simulink model "EMG_FES2-backup(14-8-2017)"  (R2014a)
settings: Solver=FixedStepDiscrete  StartTime=0.0  StopTime=100  FixedStep=1/aFES.Fs  RelTol=1e-3
InitFcn:
  | if ~exist('aFES','var')
  |   load('afes_param')
  | 
  |    aFES.Fs=1000;
  |    if (~isfield(aFES,'stimCurr'))
  |        aFES.stimCurr=[15,15];
  |    end
  |    aFES.stimFreq=25;
  |    aFES.hand='left';
  | 
  |    %set run number
  |    if (isfield(aFES,'runNum'))
  |          aFES.runNum=aFES.runNum+1;
  |    else
  |          aFES.runNum=1;
  |    end
  | 
  |    %Bias
  |    aFES.wristPosZeroBias=1.8; %e.g: goniometer reading at zeros flexion and extension
  | 
  |    %Set the upper and lower safty limit of the sensor
  |    sensorUpperSafety1=aFES.activeSensorMax+(aFES.activeSensorMax-aFES.activeSensorMin)/4 ;
  |    sensorLowerSafety1=aFES.activeSensorMin-(aFES.activeSensorMax-aFES.activeSensorMin)/4 ;
  | 
  | 
  |    %% Feedback
  |    aFES=emgfes_feedback(aFES,0,0);
  |    aFES.doubleThresh=[0.2,0.4];%Ambrosini double threshold
  | 
  |    %% FIlters
  |    [aFES.EMG_bandpass_b,aFES.EMG_bandpass_a]=butter(5,2*[40,400]/aFES.Fs);
  | 
  |    %% Tracing
  |    aFES.tracing.reflectFeedback =-1;% {1,-1} e.g if the -1, gonirmeter signal will be multiplied by -1.
  |    aFES.tracing.MaxHeightFactor=1;%when >1 scales down the max traceable height. When < 1, scales up the max traceable hieght.
  |    [~,trap_y]=trapezoid4trace();%get the trapezium to be traced
  |    n_z=5;
  |    zero_pad=zeros(n_z*aFES.Fs,1);
  | 
  |    trap_yt=[[0:1/aFES.Fs:((((n_z*aFES.Fs)+2*length(trap_y))/aFES.Fs))-(1/aFES.Fs)]', [zero_pad;trap_y;-trap_y]]; %add time to the trap
  | 
  | end
StopFcn:
  | %save the calibration data but don't apply it
  | aFES.temp.activeSensorMin=calib1_activeSensorMin;
  | aFES.temp.activeSensorMax=calib1_activeSensorMax;
  | 
  | clear calib1_activeSensorMin calib1_activeSensorMax;
  | 
  | %save(['data/afes_data_run',mat2str(aFES.runNum),'.mat'],'aFES','pw_applied','rawProcSignal');
  | save(aFES.fn,'aFES','pw_applied','rawProcSignal');
  | disp('Run data is saved');
  | 
  | disp('Calibration data is updated but not applied. ');
  | disp('To apply it run: aFES.activeSensorMin=aFES.temp.activeSensorMin;  aFES.activeSensorMax=aFES.temp.activeSensorMax; ');
  | 
  | %see if h_keepalife which is use for block event listener attachment object is present and clear it
  | if exist('h_keepalife','var')
  |         clear h_keepalife;
  | end
undefined symbols (not defined in the file or in its folder): analoginput, emgfes_feedback
libraries: dspmtrx3 x4, dspswit3 x3, simulink x2, ScienceStimHasomed_Lib x2, dspinverses x2, daqlib x1
settings Model: Creator=bethel.osuagwu  LastModifiedBy=bethel.osuagwu

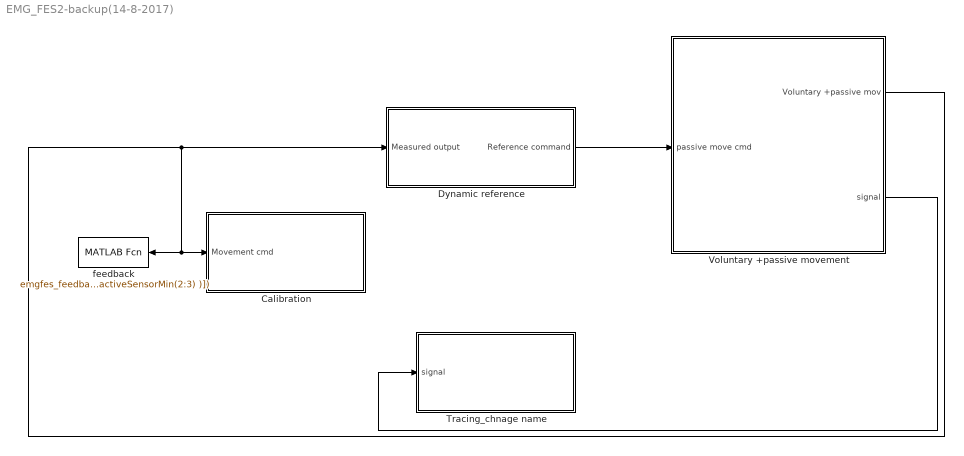
== system EMG_FES2-backup(14-8-2017) ==
  Calibration : Subsystem
  Dynamic reference : Subsystem
  Tracing_chnage name : Subsystem
  Voluntary +passive movement : Subsystem
  feedback : MATLABFcn  MATLABFcn=emgfes_feedback(aFES,[u(1), (u(2:3)'-aFES.activeSensorMin(2:3))./(aFES.activeSensorMax(2:3)-aFES.activeSensorMin(2:3) )])  OutputDimensions=0
  wires:
  Dynamic reference/1(Reference command) -> Voluntary +passive movement/1(passive move cmd)
  Voluntary +passive movement/1(Voluntary +passive mov) -> Dynamic reference/1(Measured output), feedback/1, Calibration/1(Movement cmd)
  Voluntary +passive movement/2(signal) -> Tracing_chnage name/1(signal)

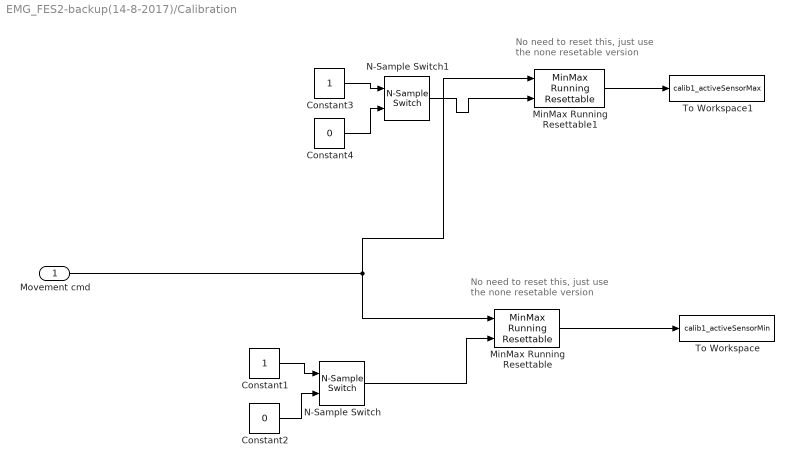
== system EMG_FES2-backup(14-8-2017)/Calibration ==
  note: No need to reset this, just use
      |  the none resetable version
  note: No need to reset this, just use
      |  the none resetable version
  Movement cmd : Inport
  Constant1 : Constant
  Constant2 : Constant  Value=0
  Constant3 : Constant
  Constant4 : Constant  Value=0
  MinMax Running Resettable : simulink/Math Operations/MinMax Running Resettable  Function=min  vinit=inf
  MinMax Running Resettable1 : simulink/Math Operations/MinMax Running Resettable  Function=max  vinit=-inf
  N-Sample Switch : dspswit3/N-Sample Switch  N=10000  reset=off  TriggerType=Rising edge  Ts=-1
  N-Sample Switch1 : dspswit3/N-Sample Switch  N=10000  reset=off  TriggerType=Rising edge  Ts=-1
  To Workspace : ToWorkspace  VariableName=calib1_activeSensorMin  SampleTime=-1
      settings: MaxDataPoints=1
  To Workspace1 : ToWorkspace  VariableName=calib1_activeSensorMax  SampleTime=-1
      settings: MaxDataPoints=1
  wires:
  N-Sample Switch1/1 -> MinMax Running Resettable1/2
  Constant1/1 -> N-Sample Switch/1
  MinMax Running Resettable1/1 -> To Workspace1/1
  MinMax Running Resettable/1 -> To Workspace/1
  N-Sample Switch/1 -> MinMax Running Resettable/2
  Constant2/1 -> N-Sample Switch/2
  Constant3/1 -> N-Sample Switch1/1
  Constant4/1 -> N-Sample Switch1/2
  Movement cmd/1 -> MinMax Running Resettable1/1, MinMax Running Resettable/1

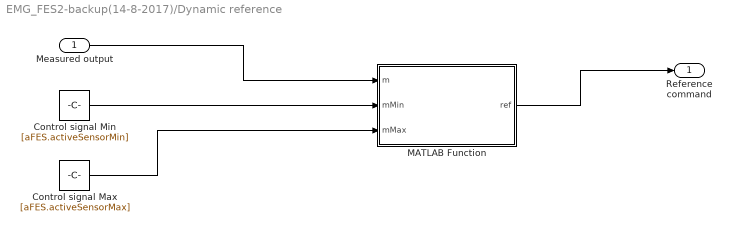
== system EMG_FES2-backup(14-8-2017)/Dynamic reference ==
  Measured output : Inport
  Control signal Max : Constant  Value=[aFES.activeSensorMax]
  Control signal Min : Constant  Value=[aFES.activeSensorMin]
  MATLAB Function : MATLAB Function  TreatAsAtomicUnit=on
  Reference command : Outport
  wires:
  Measured output/1 -> MATLAB Function/1(m)
  MATLAB Function/1(ref) -> Reference command/1
  Control signal Min/1 -> MATLAB Function/2(mMin)
  Control signal Max/1 -> MATLAB Function/3(mMax)

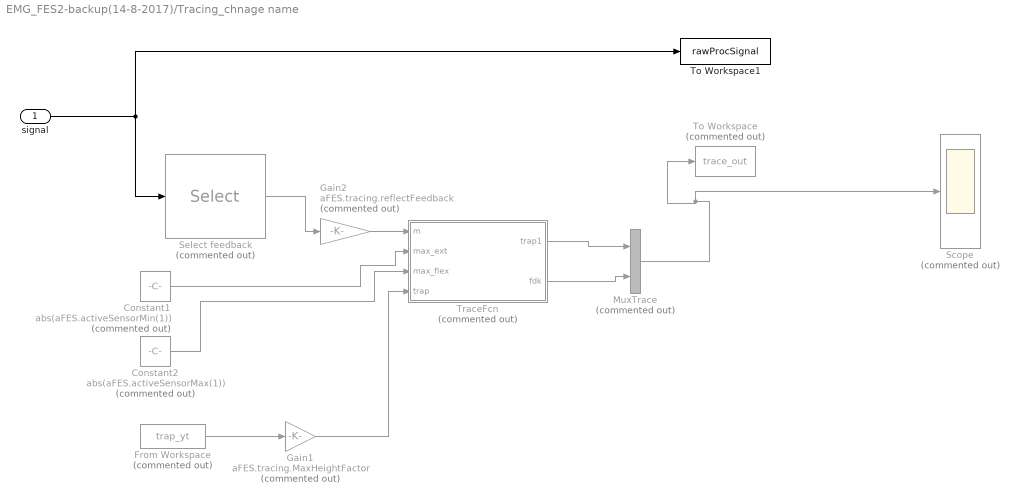
== system EMG_FES2-backup(14-8-2017)/Tracing_chnage name ==
  signal : Inport
  Constant1 : Constant  Commented=on  Value=abs(aFES.activeSensorMin(1))
  Constant2 : Constant  Commented=on  Value=abs(aFES.activeSensorMax(1))
  From Workspace : FromWorkspace  Commented=on  VariableName=trap_yt  SampleTime=1/aFES.Fs  OutputAfterFinalValue=Setting to zero
  Gain1 : Gain  Commented=on  Gain=aFES.tracing.MaxHeightFactor
  Gain2 : Gain  Commented=on  Gain=aFES.tracing.reflectFeedback
  MuxTrace : Mux  Commented=on  Inputs=2
  Scope : Scope  Commented=on
      settings: TimeRange=100  YMin=-2.25  YMax=2  SaveName=ScopeData2
  Select feedback : Selector  Commented=on  InputPortWidth=9  Indices=[7]
  To Workspace : ToWorkspace  Commented=on  VariableName=trace_out  SampleTime=-1
  To Workspace1 : ToWorkspace  VariableName=rawProcSignal  SampleTime=-1
  TraceFcn : MATLAB Function  Commented=on  TreatAsAtomicUnit=on
  wires:
  TraceFcn/1(trap1) -> MuxTrace/1
  MuxTrace/1 -> Scope/1, To Workspace/1
  Gain1/1 -> TraceFcn/4(trap)
  Constant1/1 -> TraceFcn/2(max_ext)
  Constant2/1 -> TraceFcn/3(max_flex)
  signal/1 -> Select feedback/1, To Workspace1/1
  From Workspace/1 -> Gain1/1
  TraceFcn/2(fdk) -> MuxTrace/2
  Select feedback/1 -> Gain2/1
  Gain2/1 -> TraceFcn/1(m)

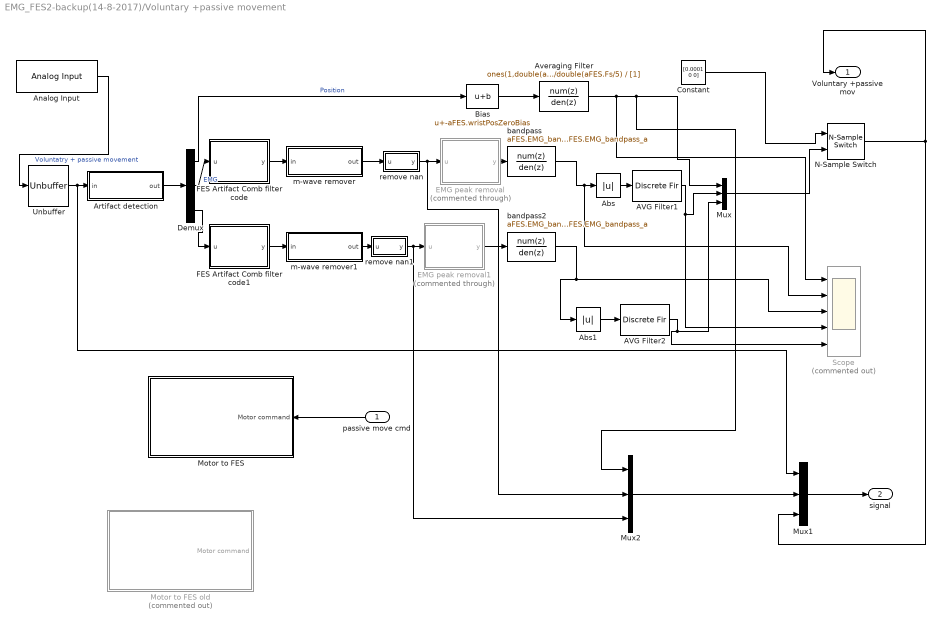
== system EMG_FES2-backup(14-8-2017)/Voluntary +passive movement ==
  passive move cmd : Inport
  " AVG Filter1" : DiscreteFir  Coefficients=ones(1,1000)/1000
  " AVG Filter2" : DiscreteFir  Coefficients=ones(1,1000)/1000
  Abs : Abs
  Abs1 : Abs
  Analog Input : daqlib/Analog Input  AcqMode=0  DeviceMenu=nidaq Dev1 (USB-6341 (BNC))  Device=nidaq Dev1 (USB-6341 (BNC))  ObjConstructor=analoginput('nidaq','Dev1')  SampleRate=1000  ActualRate=1000  SamplesPerFrame=2  InputType=Differential  NChannelsSelected=3  Channels=1$0$$2$#1$1$$2$#1$2$$2$#0$3$$1$#0$4$$1$#0$5$$1$#0$6$$1$#0$7$$1$#  NPorts=1 for all hardware channels  DataType=double
      settings: SignalType=Sample-based
  Artifact detection : Subsystem
  Averaging Filter : DiscreteFilter  Numerator=ones(1,double(aFES.Fs/5))/double(aFES.Fs/5)  Denominator=[1]
  Bias : Bias  Bias=-aFES.wristPosZeroBias
  Constant : Constant  Value=[0.0001 0 0]
  Demux : Demux  Outputs=3
  EMG peak removal : MATLAB Function  Commented=through  TreatAsAtomicUnit=on
  EMG peak removal1 : MATLAB Function  Commented=through  TreatAsAtomicUnit=on
  FES Artifact Comb filter code : MATLAB Function  TreatAsAtomicUnit=on
  FES Artifact Comb filter code1 : MATLAB Function  TreatAsAtomicUnit=on
  Motor to FES : Subsystem
  Motor to FES old : Subsystem  Commented=on
  Mux : Mux  Inputs=3
  Mux1 : Mux  Inputs=3
  Mux2 : Mux  Inputs=3
  N-Sample Switch : dspswit3/N-Sample Switch  N=10  reset=off  TriggerType=Rising edge  Ts=-1
  Scope : Scope  Commented=on  NumInputPorts=5
      settings: YMin=-1~-0.05~-0.075~0~0  YMax=0.75~0.05~0.075~0.007~0.0125
  Unbuffer : Unbuffer  SampleBasedProcessing=Same as frame based
  bandpass : DiscreteFilter  Numerator=aFES.EMG_bandpass_b  Denominator=aFES.EMG_bandpass_a
  bandpass2 : DiscreteFilter  Numerator=aFES.EMG_bandpass_b  Denominator=aFES.EMG_bandpass_a
  m-wave remover : Subsystem
  m-wave remover1 : Subsystem
  remove nan : MATLAB Function  TreatAsAtomicUnit=on
  remove nan1 : MATLAB Function  TreatAsAtomicUnit=on
  Voluntary +passive mov : Outport
  signal : Outport  Port=2
  wires:
  Analog Input/1 -> Unbuffer/1  "Voluntatry + passive movement"
  Demux/1 -> Bias/1  "Position"
  Abs/1 -> " AVG Filter1"/1
  " AVG Filter1"/1 -> Scope/4, Mux/2
  passive move cmd/1 -> Motor to FES/1(Motor command)
  Demux/2 -> FES Artifact Comb filter code/1(u)  "EMG"
  Constant/1 -> N-Sample Switch/1
  N-Sample Switch/1 -> Mux1/3, Voluntary +passive mov/1
  Unbuffer/1 -> Mux1/1, Artifact detection/1(in)
  Bias/1 -> Averaging Filter/1
  Averaging Filter/1 -> Scope/1, Mux2/1, Mux/1
  Abs1/1 -> " AVG Filter2"/1
  " AVG Filter2"/1 -> Scope/5, Mux/3
  Demux/3 -> FES Artifact Comb filter code1/1(u)
  FES Artifact Comb filter code/1(y) -> m-wave remover/1(in)
  EMG peak removal1/1(y) -> bandpass2/1
  Mux/1 -> N-Sample Switch/2
  Artifact detection/1(out) -> Demux/1
  m-wave remover/1(out) -> remove nan/1(u)
  FES Artifact Comb filter code1/1(y) -> m-wave remover1/1(in)
  EMG peak removal/1(y) -> bandpass/1
  bandpass/1 -> Scope/2, Abs/1
  bandpass2/1 -> Abs1/1, Scope/3
  remove nan/1(y) -> Mux2/2, EMG peak removal/1(u)
  remove nan1/1(y) -> Mux2/3, EMG peak removal1/1(u)
  m-wave remover1/1(out) -> remove nan1/1(u)
  Mux1/1 -> signal/1
  Mux2/1 -> Mux1/2

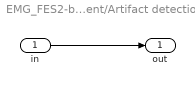
== system EMG_FES2-backup(14-8-2017)/Voluntary +passive movement/Artifact detection ==
  in : Inport
  out : Outport
  wires:
  in/1 -> out/1

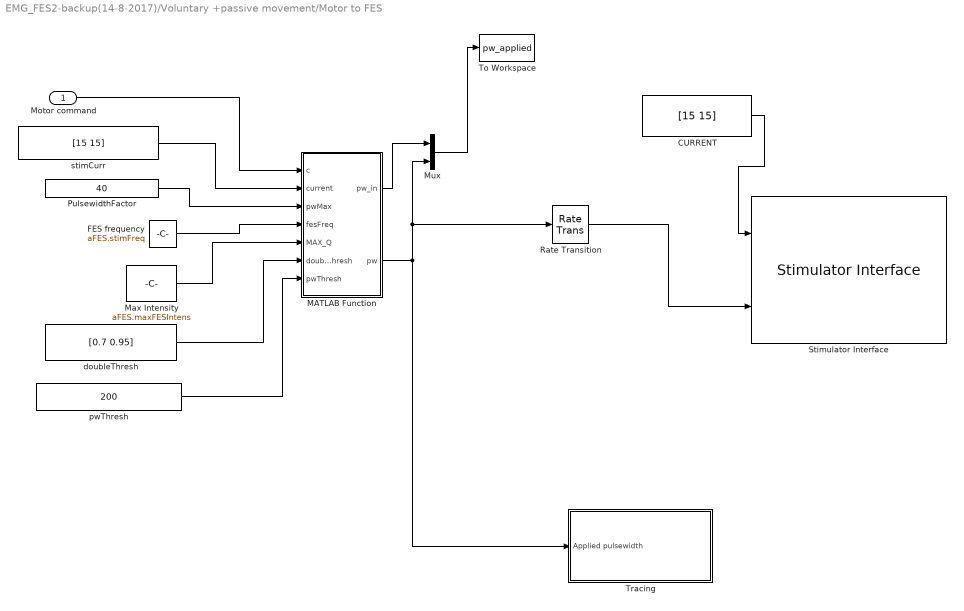
== system EMG_FES2-backup(14-8-2017)/Voluntary +passive movement/Motor to FES ==
  Motor command : Inport
  CURRENT : Constant  Value=[15 15]
  FES frequency : Constant  Value=aFES.stimFreq
  MATLAB Function : MATLAB Function  TreatAsAtomicUnit=on
  Max Intensity : Constant  Value=aFES.maxFESIntens
  Mux : Mux  Inputs=2
  PulsewidthFactor : Constant  Value=40
  Rate Transition : RateTransition
  Stimulator Interface : ScienceStimHasomed_Lib/Stimulator Interface  Ts=33/aFES.Fs  com_port=COM9  channelstim=[1,2]  tsone=round((1/aFES.stimFreq)*1000)  tstwo=5  channellf=[]  nfactor=[]  outflag=off  dtflag=off
  To Workspace : ToWorkspace  VariableName=pw_applied  SampleTime=-1
  Tracing : Subsystem
  doubleThresh : Constant  Value=[0.7 0.95]
  pwThresh : Constant  Value=200
  stimCurr : Constant  Value=[15 15]
  wires:
  CURRENT/1 -> Stimulator Interface/1
  Motor command/1 -> MATLAB Function/1(c)
  MATLAB Function/2(pw) -> Tracing/1(Applied pulsewidth), Mux/2, Rate Transition/1
  Rate Transition/1 -> Stimulator Interface/2
  stimCurr/1 -> MATLAB Function/2(current)
  Max Intensity/1 -> MATLAB Function/5(MAX_Q)
  doubleThresh/1 -> MATLAB Function/6(doubleThresh)
  MATLAB Function/1(pw_in) -> Mux/1
  Mux/1 -> To Workspace/1
  pwThresh/1 -> MATLAB Function/7(pwThresh)
  FES frequency/1 -> MATLAB Function/4(fesFreq)
  PulsewidthFactor/1 -> MATLAB Function/3(pwMax)

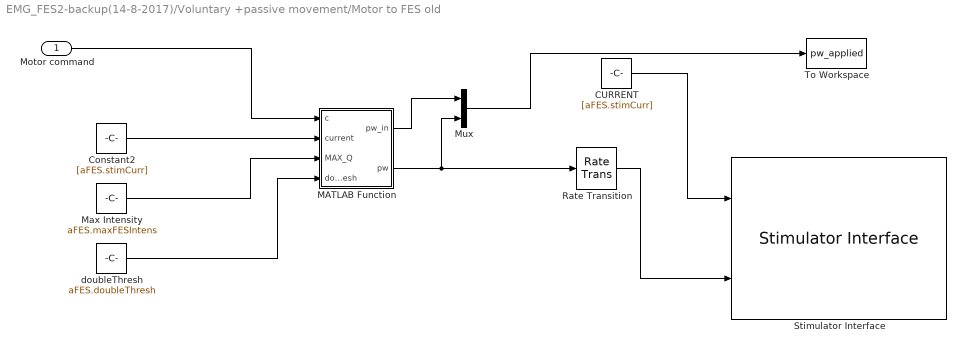
== system EMG_FES2-backup(14-8-2017)/Voluntary +passive movement/Motor to FES old ==
  Motor command : Inport
  CURRENT : Constant  Value=[aFES.stimCurr]
  Constant2 : Constant  Value=[aFES.stimCurr]
  MATLAB Function : MATLAB Function  TreatAsAtomicUnit=on
  Max Intensity : Constant  Value=aFES.maxFESIntens
  Mux : Mux  Inputs=2
  Rate Transition : RateTransition
  Stimulator Interface : ScienceStimHasomed_Lib/Stimulator Interface  Ts=33/aFES.Fs  com_port=COM9  channelstim=[1,2]  tsone=round((1/aFES.stimFreq)*1000)  tstwo=5  channellf=[]  nfactor=[]  outflag=off  dtflag=off
  To Workspace : ToWorkspace  VariableName=pw_applied  SampleTime=-1
  doubleThresh : Constant  Value=aFES.doubleThresh
  wires:
  Mux/1 -> To Workspace/1
  MATLAB Function/1(pw_in) -> Mux/1
  doubleThresh/1 -> MATLAB Function/4(doubleThresh)
  Max Intensity/1 -> MATLAB Function/3(MAX_Q)
  Constant2/1 -> MATLAB Function/2(current)
  Rate Transition/1 -> Stimulator Interface/2
  MATLAB Function/2(pw) -> Rate Transition/1, Mux/2
  Motor command/1 -> MATLAB Function/1(c)
  CURRENT/1 -> Stimulator Interface/1

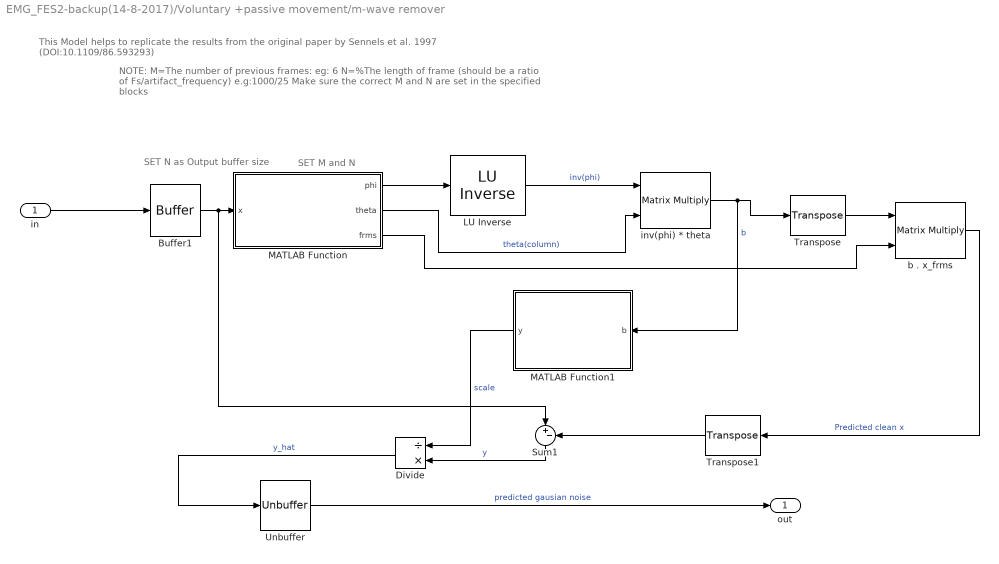
== system EMG_FES2-backup(14-8-2017)/Voluntary +passive movement/m-wave remover ==
  note: NOTE:
      | M=The number of previous frames: eg: 6
      | N=%The length of frame (should be a ratio of Fs/artifact_frequency) e.g:1000/25
      | Make sure the correct M and N are set in the specified blocks
  note: SET N as Output
      | buffer size
  note: SET M and N
  note: This Model helps to replicate the results from the original paper by Sennels et al. 1997 (DOI:10.1109/86.593293)
  in : Inport
  " LU Inverse" : dspinverses/ LU Inverse
  Buffer1 : Buffer  N=40  TreatMby1Signals=One channel
  Divide : Product  Inputs=/*
  MATLAB Function : MATLAB Function  TreatAsAtomicUnit=on
  MATLAB Function1 : MATLAB Function  TreatAsAtomicUnit=on
  Sum1 : Sum  Inputs=|+-
  Transpose : dspmtrx3/Transpose  Hermitian=off  overflowFlag=off
  Transpose1 : dspmtrx3/Transpose  Hermitian=off  overflowFlag=off
  Unbuffer : Unbuffer  SampleBasedProcessing=Same as frame based
  b . x_frms : Product  Multiplication=Matrix(*)
  inv(phi) * theta : Product  Multiplication=Matrix(*)
  out : Outport
  wires:
  Buffer1/1 -> Sum1/1, MATLAB Function/1(x)
  MATLAB Function/1(phi) -> " LU Inverse"/1
  MATLAB Function/2(theta) -> inv(phi) * theta/2  "theta(column)"
  " LU Inverse"/1 -> inv(phi) * theta/1  "inv(phi)"
  inv(phi) * theta/1 -> MATLAB Function1/1(b), Transpose/1  "b"
  Unbuffer/1 -> out/1  "predicted gausian noise"
  MATLAB Function/3(frms) -> b . x_frms/2
  Transpose/1 -> b . x_frms/1
  b . x_frms/1 -> Transpose1/1  "Predicted clean x"
  Transpose1/1 -> Sum1/2
  Sum1/1 -> Divide/2  "y"
  MATLAB Function1/1(y) -> Divide/1  "scale"
  Divide/1 -> Unbuffer/1  "y_hat"
  in/1 -> Buffer1/1

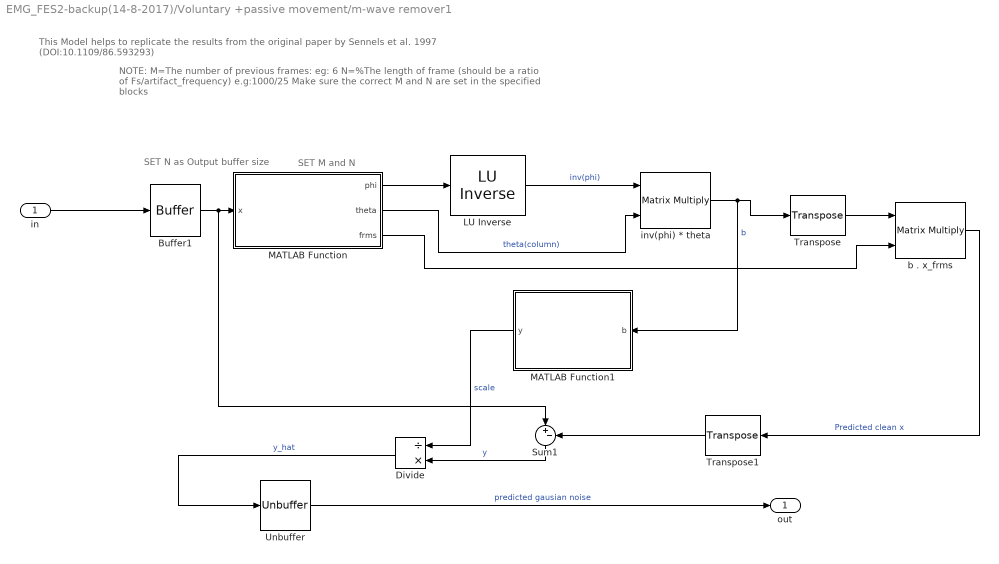
== system EMG_FES2-backup(14-8-2017)/Voluntary +passive movement/m-wave remover1 ==
  note: NOTE:
      | M=The number of previous frames: eg: 6
      | N=%The length of frame (should be a ratio of Fs/artifact_frequency) e.g:1000/25
      | Make sure the correct M and N are set in the specified blocks
  note: SET N as Output
      | buffer size
  note: SET M and N
  note: This Model helps to replicate the results from the original paper by Sennels et al. 1997 (DOI:10.1109/86.593293)
  in : Inport
  " LU Inverse" : dspinverses/ LU Inverse
  Buffer1 : Buffer  N=80  TreatMby1Signals=One channel
  Divide : Product  Inputs=/*
  MATLAB Function : MATLAB Function  TreatAsAtomicUnit=on
  MATLAB Function1 : MATLAB Function  TreatAsAtomicUnit=on
  Sum1 : Sum  Inputs=|+-
  Transpose : dspmtrx3/Transpose  Hermitian=off  overflowFlag=off
  Transpose1 : dspmtrx3/Transpose  Hermitian=off  overflowFlag=off
  Unbuffer : Unbuffer  SampleBasedProcessing=Same as frame based
  b . x_frms : Product  Multiplication=Matrix(*)
  inv(phi) * theta : Product  Multiplication=Matrix(*)
  out : Outport
  wires:
  Buffer1/1 -> Sum1/1, MATLAB Function/1(x)
  MATLAB Function/1(phi) -> " LU Inverse"/1
  MATLAB Function/2(theta) -> inv(phi) * theta/2  "theta(column)"
  " LU Inverse"/1 -> inv(phi) * theta/1  "inv(phi)"
  inv(phi) * theta/1 -> MATLAB Function1/1(b), Transpose/1  "b"
  Unbuffer/1 -> out/1  "predicted gausian noise"
  MATLAB Function/3(frms) -> b . x_frms/2
  Transpose/1 -> b . x_frms/1
  b . x_frms/1 -> Transpose1/1  "Predicted clean x"
  Transpose1/1 -> Sum1/2
  Sum1/1 -> Divide/2  "y"
  MATLAB Function1/1(y) -> Divide/1  "scale"
  Divide/1 -> Unbuffer/1  "y_hat"
  in/1 -> Buffer1/1

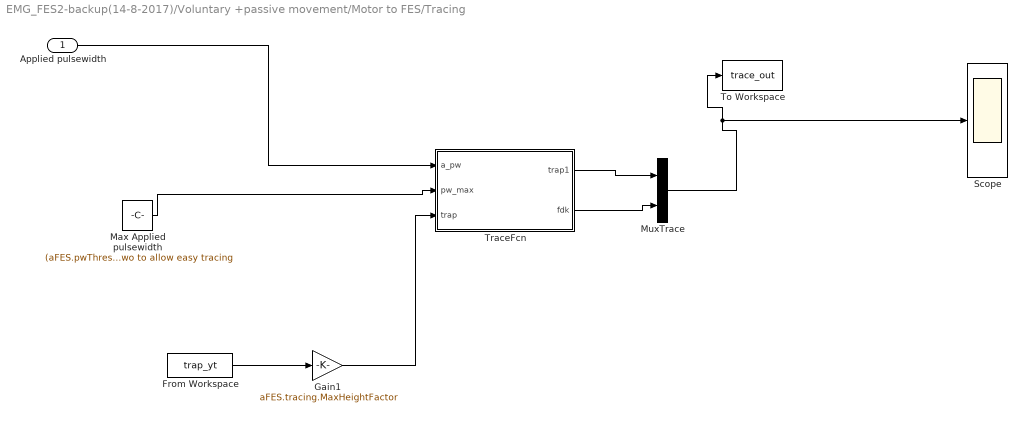
== system EMG_FES2-backup(14-8-2017)/Voluntary +passive movement/Motor to FES/Tracing ==
  Applied pulsewidth : Inport
  From Workspace : FromWorkspace  VariableName=trap_yt  SampleTime=1/aFES.Fs  OutputAfterFinalValue=Setting to zero
  Gain1 : Gain  Gain=aFES.tracing.MaxHeightFactor
  Max Applied pulsewidth : Constant  Value=(aFES.pwThresh+aFES.pwFactor*max(aFES.activeSensorMax(2:3)))/2 %we devide by two to allow easy tracing
  MuxTrace : Mux  Inputs=2
  Scope : Scope
      settings: TimeRange=100  YMin=-2.25  YMax=2  SaveName=ScopeData2
  To Workspace : ToWorkspace  VariableName=trace_out  SampleTime=-1
  TraceFcn : MATLAB Function  TreatAsAtomicUnit=on
  wires:
  TraceFcn/1(trap1) -> MuxTrace/1
  MuxTrace/1 -> To Workspace/1, Scope/1
  Gain1/1 -> TraceFcn/3(trap)
  Max Applied pulsewidth/1 -> TraceFcn/2(pw_max)
  From Workspace/1 -> Gain1/1
  TraceFcn/2(fdk) -> MuxTrace/2
  Applied pulsewidth/1 -> TraceFcn/1(a_pw)

== matlab function EMG_FES2-backup(14-8-2017)/Dynamic reference/MATLAB Function ==
  data: m input; mMin input; ref output; mMax input
function ref   = fcn(m,mMin,mMax)
%#codegen
%m(1)=position/force, extension should have negative values while flexion
%have positiove values and 0 is neutral
%m(2:3) measure of ext. EMG and Flex EMG power respectively (i.e.
%m(3)->extension and m(3)->flexion
%
%mMin and mMax are the calibration min and max resp. for m values
%
%
%
%SeSsions maked as modules can be removed without causing too much harm to
%the system, removing them just removes their minor function which does not
%affect the main system
%
%
persistent t_blocking ref_mem act_chnl_mem act_mem;
% act_chnl_mem ={0:3}. Tells us which 'vitual' channel is on. 0:none;
% 1:extension; 2:flexion; 3:tenodesis grip; 4:tenodesis release; 5:both
% flexion and extension

%assert(m<=3);

%% General parameters 

%These should be determin at the starte of every test and should be input to the fucntion
mMaxVolPercent=[1;0.9999999;0.999999];%The percentage of max voluntary value to be used as the actuall Max. E.g 0.5, means  50% of mMax is used as the actual mMax while a value of 1 means to use full mMax as mMax
mMax_=mMax.*mMaxVolPercent;%Rescale mMax

wristMax=mMax_(1);
wristMin=mMin(1);

pFlexRefMax=mMax_(3);
pFlexRefMin=mMin(3);

pExtRefMax=mMax_(2);
pExtRefMin=mMin(2);

tenodesisON=[0;0];%1=allow tenodesis; 0=No tenodesis: tenodesisON(1) for tenodesis grip. tenodesisON(2) for tenodesis release

wristExtTenoPerc =0.95;% The percentage of max wrist extension at which forced(i.e based only on wrist) tenodesis grip should be activated
wristFlexTenoPerc =0.97;%The percentage of max wrist flexion at which forced (i.e based only on wrist) tenodesis release should be activated

extTenoPerc =0.80;% The percentage of max wrist extension at which activated(i.e based on both finger and wrist, Tenodesis proper) tenodesis grip should be activated
flexTenoPerc =0.80;%The percentage of max wrist flexion at which activated (i.e based on both finger and wrist Tenodesis proper) tenodesis release should be activated

act_opposeLowerPerc=0.7;%{1= no lowering of activation threshold, 0=lower activation threshold to zero}the percentage to lower the activation of an opposing movement to give it a chance to activate

%calculate the activation threshold as a set percentage above the the
%minimun signal
act_thresh_ext=mMin(2)+0.05*mMin(2);
act_thresh_flex=mMin(3)+0.05*mMin(3);

%%Add small activation based on goniometer position. BUT FOR BETTER CONTROL, TURN THIS OFF IF
%%FES INTENSITY IS HIGH TO PRODUCE LARGE MOVEMENT \KODE*~#1.
wristActSuppON=[0;0];%{see \KODE *~#1)true to turn ON supplimentary activation when the wrist is moved above threshold:: wristActSuppON(1)=>ext; wristActSuppON(2)=>flex
wristActThresh =[wristMin;wristMax]*0.05; %the activation threshold for wrist movement

%Blocking window
oppositeRefracWin =1000;%The number of samples for which to refrain from imidiate opposite movement



%% Begin
if(isempty(t_blocking))    
   ref=m(2:3);%Make the current reference
   ref_mem=ref;
   t_blocking=0;
   act_chnl_mem=0;
   act_mem=0;
   return;
end

%update blocking timing
if t_blocking 
    if t_blocking>=oppositeRefracWin %refractory period of samples
        t_blocking=0;
    else
        t_blocking=t_blocking+1;
    end
end


%% Compute relative power
m(3)=(m(3)-pFlexRefMin)/(pFlexRefMax-pFlexRefMin);
m(2)=(m(2)-pExtRefMin)/(pExtRefMax-pExtRefMin);



%% Compute channel selection parameters
wristFlex=0;
wristExt=0;
tenoGras=0;
tenoRelease=0;
wristActSupp=[0;0];
if m(1)>0 
    wristFlex=1;%flex
    act_thresh_ext=act_thresh_ext*act_opposeLowerPerc;% lower the activation threshold of extension when the wrist is flex( Note that this might have been done by an external block):
    
    %%wrist position adds a bit of activation for flexion
    if m(1)>wristActThresh(2) && wristActSuppON(2)
        wristActSupp(2)=m(3)*0.4+0.2;
    end
    
    if(tenodesisON(2))
        if m(1)>wristMax*wristFlexTenoPerc 
            tenoRelease=1;   
        end
    end
    
else
    wristExt=1;%extension
    act_thresh_flex=act_thresh_flex*act_opposeLowerPerc ;% lower the activation threshold of flexion when the wrist extended: (Note that this might have been done by an external block)
    
    %%wrist position adds a bit of activation for extension
    if m(1)<wristActThresh(1) && wristActSuppON(1)
        wristActSupp(1)=m(2)*0.4+0.2;
    end
    
    if m(1)<wristMin*wristExtTenoPerc %TODO: check ik if (tenodesisON(1)==1
        tenoGras=1;
    end
 
end

%% Are current values greater than their thresh hold
pFlex=0;
if m(3)>act_thresh_flex
    pFlex=1;
end

pExt=0;
if m(2)>act_thresh_ext
    pExt=1;
end


%% Classify flexion and extension
isFlex=double(m(2)<m(3));

isExt=1-isFlex;
if(wristExt && pFlex)
    %So the wrist is extended but the fingers are closing
    isFlex=1; %reinforce that flexion should be on
end
if(wristFlex && pExt)
    %so the writs is flexed but the fingers are opening
    isExt=1;%reinforce that extension should be on
end

%Total flexion
isFlex=isFlex+pFlex+wristFlex;
%Total extension
isExt=isExt+pExt+wristExt;


%% Tenodesis proper (fingers and wrists)
if (wristFlex && m(1)>wristMax*flexTenoPerc && 1.5*m(2)>m(3)) && tenodesisON(2)
    %This is another way to turn on tenodesis release
    tenoRelease=tenoRelease+1;
end

if(wristExt && m(1)<wristMin*extTenoPerc && 1.5*m(3)>m(2)) && tenodesisON(1)
    %This is another way to turn on tenodesis grip
    tenoGras=tenoGras+1;
end


%% Compute ref
if tenoGras && tenodesisON(1)%i.e Tenodesis grip
    ref=m(2:3);% +wristActSupp;
    ref(2)=ref(2) + ref(2)*tenoGras*0.5; %cheat for flexion by the magnitude of the tenoGras
    act_chnl=3; %See header for the meaning of activated channels
elseif tenoRelease && tenodesisON(2)%i.e Tenodesis release
    ref=m(2:3);%+wristActSupp;
    ref(1)=ref(1) + ref(1)*tenoRelease*0.5; %cheat for flexion by the magnitude of the tenoRelease
    act_chnl=4; %See header for the meaning of activated channels
elseif isFlex>isExt
    ref=[0;m(3)];
    ref(2)=ref(2)+wristActSupp(2);
    act_chnl=2;
elseif isExt>isFlex
    ref=[m(2);0];
    ref(1)=ref(1)+wristActSupp(1);
    act_chnl=1;
elseif isExt && isFlex && isExt==isFlex
    ref=m(2:3);%+wristActSupp;
    act_chnl=5;
else   
    ref=[0;0];
    act_chnl=0;
end
act=sum(ref);   

%% Check if we can block activation
%%implements blocking of immediate opposite movement
if ~t_blocking || act_chnl==act_chnl_mem && act>act_mem% The operator precidence here should lead to the correct operation
    t_blocking=1;% start blocking of further imidiate opposite change
else
    ref=ref_mem; 
end


%% Save to mem
if(ref(1)~=ref_mem(1) || ref(2)~=ref_mem(2))
    act_mem=act;
    act_chnl_mem=act_chnl;
    ref_mem=ref;
    
end

== matlab function EMG_FES2-backup(14-8-2017)/Voluntary +passive movement/FES Artifact Comb filter code ==
  data: u input; y output
function y  = fcn(u)
%#codegen

persistent u_mem;
fes_freq=25;%FES frequency
Fs=1000;%EMG/data samplerate
K=40;%round(Fs/fes_freq); %Comb filter order = (1/fes_freq)*Fs
a=-1;%{-1 to 0}
if isempty(u_mem)
    u_mem=zeros(K,1);
end





%% Comb filtering
% Forward comb
y=u+ a*u_mem(1);



u_mem(1:end-1)=u_mem(2:end);
u_mem(end)=u;



end





%

== matlab function EMG_FES2-backup(14-8-2017)/Voluntary +passive movement/Motor to FES/MATLAB Function ==
  data: pw_in output; c input; current input; pw output; pwMax input; fesFreq input; MAX_Q input; doubleThresh input; pwThresh input
function [pw_in,pw] = fcn(c,current,pwMax,fesFreq,MAX_Q,doubleThresh,pwThresh)
%#codegen
% c is the controller output
% current is a vector(1 ele/chnl) of FES current in milliamps
% pwMax is the max pulsewidth 
% fesFreq is the FES frequency
% MAX_Q= eg.5000;%maxmum FES intensity =current x pulsewidth *freq
% doubleThresh {[OFF thresh; ON thresh]}is the double thresh similer to that by Ambrosini
% pwThresh is the starting pulsewidth once activation reaches
%threshold
persistent  FES_ON pw_smooth;


if isempty(pw_smooth)
    %c_mem=zeros(30,2);
    FES_ON=[0;0];
    pw_smooth=[0;0];
    
end


%% (Module) Avoid spikes in Stimulation
% if false
% c(dcdt>0.5)=median(c_mem);
% %upadte memory of controller output
%  c_mem(1:end-1,:)=c_mem(2:end,:);
%  c_mem(end,:)=c;
% end

%compute pulsewidth
if(doubleThresh(2))
    pw=[0;0];
    for chni=1:2
        if FES_ON(chni) %If the channel is ON, check if it has dropped below first double thresh
            if c(chni)<doubleThresh(1)%If the channel has dropped below the first thresh, then turn it OFF
                pw(chni)=0;
                FES_ON(chni)=0;
            else %But if the channel is still above the OFF thresh, then proportionally set the pw
                %pw(chni)=200+c(chni)*30;%
                pw(chni)=pwThresh+c(chni)*pwMax;
                FES_ON(chni)=1;
            end
        else %But is the channel currently OFF, Check if it has activation above ON thresh
            if c(chni)>doubleThresh(2)% If the activation is above ON thresh,then proportionally set the pw
                %pw(chni)=200+c(chni)*30;%
                pw(chni)=pwThresh+c(chni)*pwMax;
                FES_ON(chni)=1;
            else %but if it is still under the ON thresh, make sure that it is set to off
                pw(chni)=0;
                FES_ON(chni)=0;
            end
        end
    end
    
else %Double threshold is disabled, need to proportionally set pw
    pw=(c).*pwMax;%OR %pw=pwThresh+(c).*pwMax;
    
    
    
    %pw(pw<0)=0;
    %pw(pw>50)=pw(pw>50)+10;%add a bias
    pw(pw<50)=0;
end

%% Limit max Intensity of FES
q=current.*pw*fesFreq;
q_=q>MAX_Q;
for nq=1:length(q_)
    if q_(nq)
        pw(nq)=MAX_Q/(current(nq)*fesFreq);
        'Motor to FES: limits [ch,pulsewidth_limit]'
        [nq pw(nq)]
    end
end

%% The estimated pw is essentially our input pw
pw_in=pw;% If no further modification below, then pw_in==pw


%% (Module)Controller output based change in stimulation for opposing movement assistance



%% (Module)Error based change in stimulation for opposing movement assistance


%% (Module) Smoothness controller for pw
pw_step=0.1;%(TODO: should be a function of max pw and samplerate)allowed positive step chnage per sample
pw=abs(pw_smooth+sign(pw-pw_smooth)*pw_step); %the abs here is fine as far as the step size is small(e.g <5)
%pw(pw<pw_step)=0;NOTE open this 
pw_smooth=pw;
%-----------------------------

== matlab function EMG_FES2-backup(14-8-2017)/Voluntary +passive movement/m-wave remover/MATLAB Function ==
  data: x input; phi output double; theta output; frms output
function [phi,theta,frms] = fcn(x)
%#codegen
persistent t_sample phi_mem  frms_mem ;

%General param
M=6; %The number of previous frames 
N=40; %The length of frame (should be a ratio of Fs/artifact_frequency)

% Performance parameter
freshPhi =1;% when =1:recompute phi(covariance matix) all the phi; when =0:update phi with only new values

if isempty(t_sample)
    t_sample=0;
    frms_mem=zeros(M,N);
    
    phi_mem=zeros(M,M);
end
t_sample=t_sample+1;

%make x a row vector
x=x';


%% compute phi
frms=frms_mem;
%equ 7 and 8
if(freshPhi)
    % compute phi fresh all the time
    phi=(frms*frms');
else
    %we can compute only the required column (first) and row (first)of phi
    %matrix and push the new values into phi
    phi_mem(2:end,2:end)=phi_mem(1:end-1,1:end-1);
    phi_mem(1,:)=frms(1,:)*frms';
    phi_mem(:,1)=phi_mem(1,:)';
    %phi-phi_mem
    phi=phi_mem;
end


%% compute theta
theta=(x*frms')';
%t_sample
%if t_sample==15
%    y=4;
%end


%% update frame
frms_mem(2:end,:)=frms_mem(1:end-1,:);
frms_mem(1,:)=x;

== matlab function EMG_FES2-backup(14-8-2017)/Voluntary +passive movement/FES Artifact Comb filter code1 ==
  data: u input; y output
function y  = fcn(u)
%#codegen

persistent u_mem;
fes_freq=25;%FES frequency
Fs=1000;%EMG/data samplerate
K=40;%round(Fs/fes_freq); %Comb filter order = (1/fes_freq)*Fs
a=-1;%{-1 to 0}
if isempty(u_mem)
    u_mem=zeros(K,1);
end





%% Comb filtering
% Forward comb
y=u+ a*u_mem(1);



u_mem(1:end-1)=u_mem(2:end);
u_mem(end)=u;
end





%

== matlab function EMG_FES2-backup(14-8-2017)/Voluntary +passive movement/EMG peak removal1 ==
  data: u input; y output
function y  = fcn(u)
%#codegen
%peak removal
peak_thresh=0.5;
dmdt_thresh=0.3;
blocking_win=50;
persistent u_mem t_;
if isempty(u_mem)
    u_mem=zeros(1000,1);
    t_=0;
end

if (dmdt_thresh<abs(u)-abs(u_mem(end))&& t_==0)%if the change in value to too large  then block with no stats
    t_=1;
else   
    if((abs(u)>peak_thresh || dmdt_thresh<abs(u)-abs(u_mem(end))) && t_==0) %detect high amplitude,peak, and start blocking
        if(abs(u)>std(u_mem))
            t_=1;
        end
    end

    
end


if t_
    u=0;%block
   t_=t_+1;
end
if(t_==blocking_win) %stop blocking after n samples
    t_=0; 
end

u_mem(1:end-1)=u_mem(2:end);
u_mem(end)=u;
y=u;
end





%

== matlab function EMG_FES2-backup(14-8-2017)/Voluntary +passive movement/EMG peak removal ==
  data: u input; y output
function y  = fcn(u)
%#codegen
%peak removal
peak_thresh=0.5;
dmdt_thresh=0.3;
blocking_win=50;
persistent u_mem t_;
if isempty(u_mem)
    u_mem=zeros(1000,1);
    t_=0;
end

if (dmdt_thresh<abs(u)-abs(u_mem(end))&& t_==0)%if the change in value to too large  then block with no stats
    t_=1;
else   
    if((abs(u)>peak_thresh || dmdt_thresh<abs(u)-abs(u_mem(end))) && t_==0) %detect high amplitude,peak, and start blocking
        if(abs(u)>std(u_mem))
            t_=1;
        end
    end

    
end


if t_
    u=0;%block
   t_=t_+1;
end
if(t_==blocking_win) %stop blocking after n samples
    t_=0; 
end

u_mem(1:end-1)=u_mem(2:end);
u_mem(end)=u;
y=u;
end





%

== matlab function EMG_FES2-backup(14-8-2017)/Voluntary +passive movement/remove nan ==
  data: u input; y output
function y  = fcn(u)
%#codegen

y=u;
if isnan(y)
    y=0;
end





%

== matlab function EMG_FES2-backup(14-8-2017)/Voluntary +passive movement/remove nan1 ==
  data: u input; y output
function y  = fcn(u)
%#codegen

y=u;
if isnan(y)
    y=0;
end





%

== matlab function EMG_FES2-backup(14-8-2017)/Voluntary +passive movement/m-wave remover/MATLAB Function1 ==
  data: b input; y output
function y = fcn(b)
%#codegen


y = sqrt(1+sum(b.^2));
%       OR
%y = (1+sum(b));%approximated for speed

== matlab function EMG_FES2-backup(14-8-2017)/Voluntary +passive movement/m-wave remover1/MATLAB Function ==
  data: x input; phi output double; theta output; frms output
function [phi,theta,frms] = fcn(x)
%#codegen
persistent t_sample phi_mem  frms_mem ;

%General param
M=6; %The number of previous frames 
N=80; %The length of frame (should be a ratio of Fs/artifact_frequency)

% Performance parameter
freshPhi =1;% when =1:recompute phi(covariance matix) all the phi; when =0:update phi with only new values

if isempty(t_sample)
    t_sample=0;
    frms_mem=zeros(M,N);
    
    phi_mem=zeros(M,M);
end
t_sample=t_sample+1;

%make x a row vector
x=x';


%% compute phi
frms=frms_mem;
%equ 7 and 8
if(freshPhi)
    % compute phi fresh all the time
    phi=(frms*frms');
else
    %we can compute only the required column (first) and row (first)of phi
    %matrix and push the new values into phi
    phi_mem(2:end,2:end)=phi_mem(1:end-1,1:end-1);
    phi_mem(1,:)=frms(1,:)*frms';
    phi_mem(:,1)=phi_mem(1,:)';
    %phi-phi_mem
    phi=phi_mem;
end


%% compute theta
theta=(x*frms')';
%t_sample
%if t_sample==15
%    y=4;
%end


%% update frame
frms_mem(2:end,:)=frms_mem(1:end-1,:);
frms_mem(1,:)=x;

== matlab function EMG_FES2-backup(14-8-2017)/Voluntary +passive movement/m-wave remover1/MATLAB Function1 ==
  data: b input; y output
function y = fcn(b)
%#codegen


y = sqrt(1+sum(b.^2));
%       OR
%y = (1+sum(b));%approximated for speed

== matlab function EMG_FES2-backup(14-8-2017)/Tracing_chnage name/TraceFcn ==
  data: m input; max_ext input; max_flex input; trap input; trap1 output; fdk output
function [trap1,fdk]    = fcn(m,max_ext,max_flex,trap)
%#codegen
%coder.extrinsic('plot','hold');
% persistent ts;
% if isempty(ts)
%     ts=0;
%     %m_mem=zeros(10*1000,1);
% end
%m_mem(1:end-1)=m_mem(2:end);
%m_mem(end)=m(1);

%scale extension
if(m(1)>0)
    m(1)=m(1)/max_ext;
elseif m(1)<0
    m(1)=m(1)/max_flex;
end
    
%ts=ts+1;
 trap1=trap;
 
 fdk=m(1);
 
%stopSingnal=0;
%  if(ts==length(trap))
%      stopSingnal=1;
%  end

== matlab function EMG_FES2-backup(14-8-2017)/Voluntary +passive movement/Motor to FES old/MATLAB Function ==
  data: pw_in output; c input; current input; pw output; MAX_Q input; doubleThresh input
function [pw_in,pw] = fcn(c,current,MAX_Q,doubleThresh)
%#codegen
% c is the controller output
% dcdt is the derivative of c
%MAX_Q= eg.5000;%maxmum intensity =current x pulsewidth
persistent  FES_ON pw_smooth;

pMax=300;
if isempty(pw_smooth)
    %c_mem=zeros(30,2);
    FES_ON=[0;0];
    pw_smooth=[0;0];
end


%% (Module) Avoid spikes in Stimulation
% if false
% c(dcdt>0.5)=median(c_mem);
% %upadte memory of controller output
%  c_mem(1:end-1,:)=c_mem(2:end,:);
%  c_mem(end,:)=c;
% end

%compute pulsewidth
if(doubleThresh(2))
    pw=[0;0];
    for chni=1:2
        if FES_ON(chni)
            if c(chni)<doubleThresh(1)
                pw(chni)=0;
                FES_ON(chni)=0;
            else
                pw(chni)=200+c(chni).*30;
                FES_ON(chni)=1;
            end
        else %it is currently off
            if c(chni)>doubleThresh(2)
                pw(chni)=200+c(chni).*30;
                FES_ON(chni)=1;
            else
                pw(chni)=0;
                FES_ON(chni)=0;
            end
        end
    end
    
else
    pw=(c).*pMax;
    pw(pw<0)=0;
    %pw(pw>50)=pw(pw>50)+10;%add a bias
    pw(pw<50)=0;
end

%% Limit max Intensity of FES
q=current.*pw;
q_=q>MAX_Q;
for nq=1:length(q_)
    if q_(nq)
        pw(nq)=MAX_Q/current(nq);
        'Motor to FES: limits [ch,pulsewidth_limit]'
        [nq pw(nq)]
    end
end

%% The estimated pw is essentially our input pw
pw_in=pw;% If no further modification below, then pw_in==pw


%% (Module)Controller output based change in stimulation for opposing movement assistance



%% (Module)Error based change in stimulation for opposing movement assistance


%% (Module) Smoothness controller for pw
pw_step=0.2;%(TODO: should be a function of max pw and samplerate)allowed positive step chnage per sample
pw=abs(pw_smooth+sign(pw-pw_smooth)*pw_step); %the abs here is fine as far as the step size is small(e.g <5)
%pw(pw<pw_step)=0;NOTE open this 
pw_smooth=pw;
%-----------------------------

== matlab function EMG_FES2-backup(14-8-2017)/Voluntary +passive movement/Motor to FES/Tracing/TraceFcn ==
  data: a_pw input; pw_max input; trap input; trap1 output; fdk output
function [trap1,fdk]    = fcn(a_pw,pw_max,trap)
%#codegen
%coder.extrinsic('plot','hold');
% persistent ts;
% if isempty(ts)
%     ts=0;
%     %m_mem=zeros(10*1000,1);
% end
%m_mem(1:end-1)=m_mem(2:end);
%m_mem(end)=m(1);

%scale extension
% if(m(1)>0)
    a_pw=a_pw./pw_max;
% elseif m(1)<0
%     m(1)=m(1)/max_flex;
% end
    
%ts=ts+1;
 trap1=trap;
 
 fdk=a_pw(1)-a_pw(2);%in this way the direction and magnitude of fdk tels which feedback is bigger(+ve for ED and -ve for FDS)
 
%stopSingnal=0;
%  if(ts==length(trap))
%      stopSingnal=1;
%  end
